simulink model "validation_sim"  (R2021a)
settings: Solver=VariableStepAuto  StartTime=0.0  StopTime=0.35  RelTol=1e-3
values from neighbouring files (symbols this model uses):
  tau_area = A0 / vt_inf    [get_tau_area.m]    (also in labeca_02_simulink_export.m = get_tau_area(filename); labeca_02_validacao_2.m = A0 / y_inf)
  tau_nep = 1/a    [get_tau_nep.m]    (also in labeca_02_simulink_export.m = get_tau_nep(filename); labeca_02_validacao_2.m)
undefined symbols (not defined in the file or in its folder): K
settings Model: Creator=henri  LastModifiedBy=carol

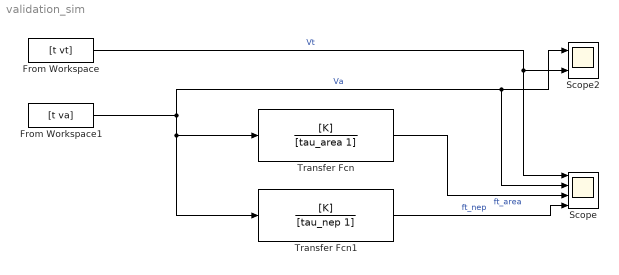
== system validation_sim ==
  From Workspace : FromWorkspace  VariableName=[t vt]  OutDataTypeStr=double
  From Workspace1 : FromWorkspace  VariableName=[t va]  OutDataTypeStr=double
  Scope : Scope  NumInputPorts=4
  Scope2 : Scope  NumInputPorts=2
  Transfer Fcn : TransferFcn  Numerator=[K]  Denominator=[tau_area 1]
  Transfer Fcn1 : TransferFcn  Numerator=[K]  Denominator=[tau_nep 1]
  wires:
  From Workspace1/1 -> Transfer Fcn1/1, Transfer Fcn/1, Scope/2, Scope2/1  "Va"
  From Workspace/1 -> Scope/1, Scope2/2  "Vt"
  Transfer Fcn/1 -> Scope/3  "ft_area"
  Transfer Fcn1/1 -> Scope/4  "ft_nep"
